simulink model "proiectv2"  (Simulink 7.4)
settings: Solver=ode23tb  StartTime=0.0  StopTime=0.1  RelTol=1e-3
libraries: powerlib x10
settings Model: Creator=Cristi  LastModifiedBy=Cristi

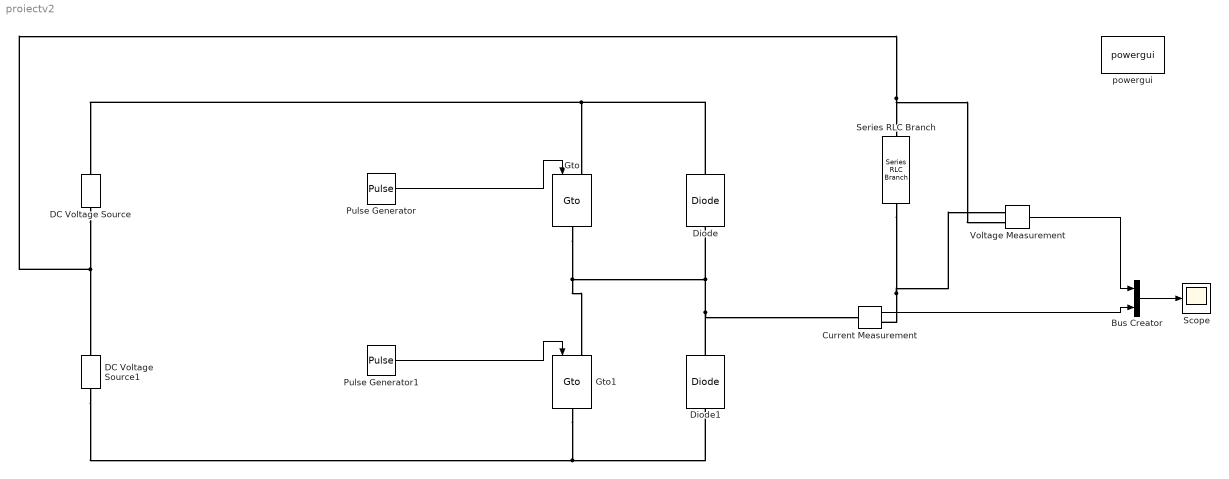
== system proiectv2 ==
  Bus Creator : BusCreator  Inputs=2
  Current Measurement : powerlib/Measurements/Current Measurement  DialogController=POWERSYS.PowerSysDialog  SystemSampleTime=-1  PhasorSimulation=off  OutputType=Complex  PSBequivalent=0
  DC Voltage Source : powerlib/Electrical Sources/DC Voltage Source  DialogController=POWERSYS.PowerSysDialog  SystemSampleTime=-1  Amplitude=115  Measurements=None
  DC Voltage Source1 : powerlib/Electrical Sources/DC Voltage Source  DialogController=POWERSYS.PowerSysDialog  SystemSampleTime=-1  Amplitude=115  Measurements=None
  Diode : powerlib/Power Electronics/Diode  DialogController=POWERSYS.PowerSysDialog  SystemSampleTime=-1  Ron=0.001  Lon=0  Vf=0.7  IC=0  UseSnubber=off  Rs=500  Cs=250e-9  Measurements=off
  Diode1 : powerlib/Power Electronics/Diode  DialogController=POWERSYS.PowerSysDialog  SystemSampleTime=-1  Ron=0.001  Lon=0  Vf=0.7  IC=0  UseSnubber=off  Rs=500  Cs=250e-9  Measurements=off
  Gto : powerlib/Power Electronics/Gto  DialogController=POWERSYS.PowerSysDialog  SystemSampleTime=-1  Ron=0.001  Lon=0  Vf=1  Tf=10e-6  Tt=20e-6  IC=0  Rs=1e5  Cs=inf  Measurements=off
  Gto1 : powerlib/Power Electronics/Gto  DialogController=POWERSYS.PowerSysDialog  SystemSampleTime=-1  Ron=0.001  Lon=0  Vf=1  Tf=10e-6  Tt=20e-6  IC=0  Rs=1e5  Cs=inf  Measurements=off
  Pulse Generator : DiscretePulseGenerator  PulseType=Time based  Amplitude=115  Period=0.02  PulseWidth=50  PhaseDelay=0  SampleTime=1
  Pulse Generator1 : DiscretePulseGenerator  PulseType=Time based  Amplitude=115  Period=0.02  PulseWidth=50  PhaseDelay=0.01  SampleTime=1
  Scope : Scope
      settings: TimeRange=0.1
  Series RLC Branch : powerlib/Elements/Series RLC Branch  DialogController=POWERSYS.PowerSysDialog  PhysicalDomain=powersysdomain  SubClassName=unknown  LeftPortType=p1  RightPortType=p1  LConnTagsString=__new0  RConnTagsString=__new0  BranchType=R  Resistance=5  Inductance=1e-3  SetiL0=off  InitialCurrent=0  Capacitance=1e-6  Setx0=off  InitialVoltage=0  Measurements=None
  Voltage Measurement : powerlib/Measurements/Voltage Measurement  DialogController=POWERSYS.PowerSysDialog  SystemSampleTime=-1  PhasorSimulation=off  OutputType=Complex  PSBequivalent=0
  powergui : powerlib/powergui  Priority=1  SystemSampleTime=-1  SimulationMode=Continuous  SampleTime=50e-6  frequency=60  SPID=off  DisableSnubberDevices=off  DisableRonSwitches=off  DisableVfSwitches=off  SwTol=0  Interpol=off  frequencyindice=0  echomessages=off  HookPort=off  DisplayEquations=off  FunctionMessages=off  EnableUseOfTLC=off  x0status=blocks  RestoreLinks=warning  Frange=[0:2:500]  Ylog=off  Xlog=on  ShowGrid=off  save=off  variable=ZData  ZoomFFT=on  StartTime=0.0  cycles=1  DisplayStyle=1  fundamental=60  FreqAxis=off  MaxFrequency=1000  frequencyindicesteady=1  RmsSteady=1  display=off  Ts=0  methode=off
  wires:
  Pulse Generator1/1 -> Gto1/1
  Pulse Generator/1 -> Gto/1
  Bus Creator/1 -> Scope/1
  Current Measurement/1 -> Bus Creator/2
  Voltage Measurement/1 -> Bus Creator/1
  connections:
  DC Voltage Source/LConn1 -- DC Voltage Source1/RConn1 -- Series RLC Branch/LConn1 -- Voltage Measurement/LConn2
  DC Voltage Source1/LConn1 -- Diode1/LConn1 -- Gto1/RConn1
  Diode/RConn1 -- DC Voltage Source/RConn1 -- Gto/LConn1
  Diode1/RConn1 -- Gto/RConn1 -- Gto1/LConn1 -- Diode/LConn1 -- Current Measurement/LConn1
  Series RLC Branch/RConn1 -- Current Measurement/RConn1 -- Voltage Measurement/LConn1
